simulink model "mdl"  (R2020b)
settings: Solver=VariableStepAuto  StartTime=0.0  StopTime=20.0  RelTol=1e-3
settings Model: Creator=mluser  LastModifiedBy=mluser

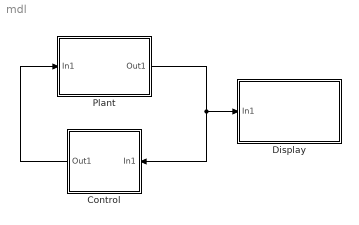
== system mdl ==
  Control : Subsystem
  Display : Subsystem
  Plant : Subsystem
  wires:
  Plant/1(Out1) -> Display/1(In1), Control/1(In1)
  Control/1(Out1) -> Plant/1(In1)

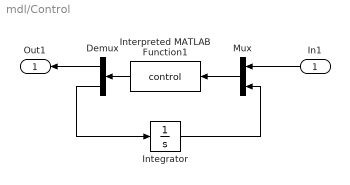
== system mdl/Control ==
  In1 : Inport
  Demux : Demux  Outputs=2
  Integrator : Integrator
  Interpreted MATLAB Function1 : MATLABFcn  MATLABFcn=control
  Mux : Mux  Inputs=2
  Out1 : Outport
  wires:
  Interpreted MATLAB Function1/1 -> Demux/1
  Demux/1 -> Out1/1
  Demux/2 -> Integrator/1
  In1/1 -> Mux/1
  Integrator/1 -> Mux/2
  Mux/1 -> Interpreted MATLAB Function1/1

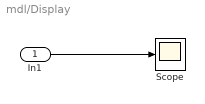
== system mdl/Display ==
  In1 : Inport
  Scope : Scope
  wires:
  In1/1 -> Scope/1

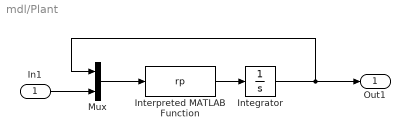
== system mdl/Plant ==
  In1 : Inport
  Integrator : Integrator  InitialCondition=1
  Interpreted MATLAB Function : MATLABFcn  MATLABFcn=rp
  Mux : Mux  Inputs=2
  Out1 : Outport
  wires:
  Interpreted MATLAB Function/1 -> Integrator/1
  Mux/1 -> Interpreted MATLAB Function/1
  Integrator/1 -> Mux/1, Out1/1
  In1/1 -> Mux/2
